simulink model "DDC_test"  (Simulink 7.4)
settings: Solver=ode3  StartTime=0.0  StopTime=Inf  FixedStep=1  RelTol=1e-3
undefined symbols (not defined in the file): Fs, get, j, sided, Two
libraries: simulink x6, dspsnks4 x5, dspsigops x2
settings Model: Creator=babjak  LastModifiedBy=babjak

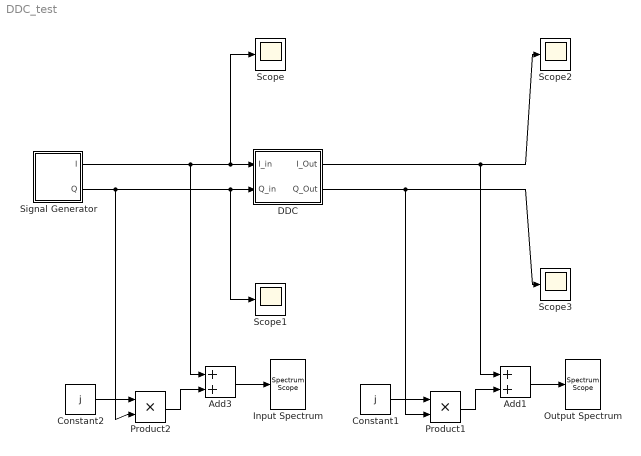
== system DDC_test ==
  Add1 : Sum  OutDataType=fixdt(1, 16)  OutScaling=2^-10
  Add3 : Sum  OutDataType=fixdt(1, 16)  OutScaling=2^-10
  Constant1 : Constant  Value=j  OutDataType=fixdt(1, 16)  OutScaling=2^0
  Constant2 : Constant  Value=j  OutDataType=fixdt(1, 16)  OutScaling=2^0
  DDC : Subsystem
  Input Spectrum : dspsnks4/Spectrum Scope  DialogController=dspdialog.SpectrumScope  DialogControllerArgs=DataTag3  SystemSampleTime=-1  ScopeProperties=on  Domain=Frequency  HorizSpan=1  UseBuffer=on  BufferSize=128  Overlap=0  inpFftLenInherit=off  FFTlength=128  numAvg=2  DisplayProperties=off  AxisGrid=on  Memory=off  FrameNumber=on  AxisLegend=off  AxisZoom=off  OpenScopeAtSimStart=on  OpenScopeImmediately=off  FigPos=get(0,'defaultfigureposition')  AxisProperties=off  XUnits=Hertz  XRange=Two-sided ((-Fs/2...Fs/2])  XDisplay=0  InheritXIncr=off  XIncr=3.6e-7  XLabel=Samples  XLimit=Auto  YUnits=dBW/Hertz  XMax=1  XMin=0  YLabel=Magnitude-squared, dB  LineProperties=off  wintypeSpecScope=Boxcar  RsSpecScope=50  betaSpecScope=5  winsampSpecScope=Periodic  XAxisParamsVer=6.9
      settings: YMin=-10  YMax=10
  Output Spectrum : dspsnks4/Spectrum Scope  DialogController=dspdialog.SpectrumScope  DialogControllerArgs=DataTag4  SystemSampleTime=-1  ScopeProperties=on  Domain=Frequency  HorizSpan=1  UseBuffer=on  BufferSize=128  Overlap=0  inpFftLenInherit=off  FFTlength=128  numAvg=2  DisplayProperties=off  AxisGrid=on  Memory=off  FrameNumber=on  AxisLegend=off  AxisZoom=off  OpenScopeAtSimStart=on  OpenScopeImmediately=off  FigPos=get(0,'defaultfigureposition')  AxisProperties=off  XUnits=Hertz  XRange=Two-sided ((-Fs/2...Fs/2])  XDisplay=0  InheritXIncr=off  XIncr=1.44e-6  XLabel=Samples  XLimit=Auto  YUnits=dBW/Hertz  XMax=1  XMin=0  YLabel=Magnitude-squared, dB  LineProperties=off  wintypeSpecScope=Boxcar  RsSpecScope=50  betaSpecScope=5  winsampSpecScope=Periodic  XAxisParamsVer=6.9
      settings: YMin=-10  YMax=10
  Product1 : Product  OutDataType=fixdt(1, 16)  OutScaling=2^0  RndMeth=Zero
  Product2 : Product  OutDataType=fixdt(1, 16)  OutScaling=2^0  RndMeth=Zero
  Scope{,1..3} (4 alike) : Scope
      Scope2 settings: SaveName=ScopeData2
      Scope3 settings: SaveName=ScopeData3
  Signal Generator : Subsystem
  wires:
  DDC/1(I_Out) -> Scope2/1, Add1/1
  DDC/2(Q_Out) -> Scope3/1, Product1/2
  Signal Generator/1(I) -> DDC/1(I_in), Scope/1, Add3/1
  Signal Generator/2(Q) -> DDC/2(Q_in), Scope1/1, Product2/2
  Constant2/1 -> Product2/1
  Product2/1 -> Add3/2
  Add3/1 -> Input Spectrum/1
  Constant1/1 -> Product1/1
  Product1/1 -> Add1/2
  Add1/1 -> Output Spectrum/1

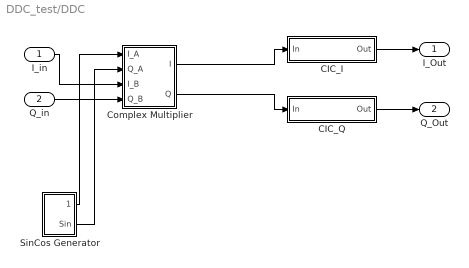
== system DDC_test/DDC ==
  I_in : Inport  DataType=Specify via dialog  OutDataType=fixdt(1,14,0)  OutDataTypeStr=fixdt(1,14,0)
  Q_in : Inport  Port=2  DataType=Specify via dialog  OutDataType=fixdt(1,14,0)  OutDataTypeStr=fixdt(1,14,0)
  CIC_I : Subsystem
  CIC_Q : Subsystem
  Complex Multiplier : Subsystem
  SinCos Generator : Subsystem
  I_Out : Outport
  Q_Out : Outport  Port=2
  wires:
  SinCos Generator/1(Cos) -> Complex Multiplier/1(I_A)
  SinCos Generator/2(Sin) -> Complex Multiplier/2(Q_A)
  Complex Multiplier/1(I) -> CIC_I/1(In)
  I_in/1 -> Complex Multiplier/3(I_B)
  Complex Multiplier/2(Q) -> CIC_Q/1(In)
  Q_in/1 -> Complex Multiplier/4(Q_B)
  CIC_I/1(Out) -> I_Out/1
  CIC_Q/1(Out) -> Q_Out/1

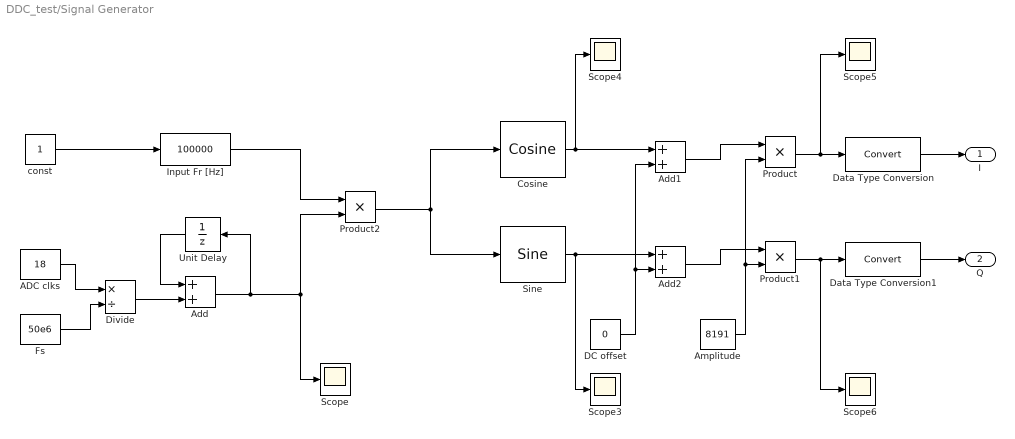
== system DDC_test/Signal Generator ==
  ADC clks : Constant  Value=18  OutDataTypeMode=double  OutDataType=fixdt(1,16)  ConRadixGroup=Best Precision: Vector-wise  OutDataTypeStr=double  SampleTime=Inf
  Add : Sum  OutDataTypeMode=double  OutDataTypeStr=double  SampleTime=1
  Add1 : Sum  OutDataType=fixdt(1, 16)  OutScaling=2^-10
  Add2 : Sum  OutDataType=fixdt(1, 16)  OutScaling=2^-10
  Amplitude : Constant  Value=8191  OutDataType=fixdt(1, 16)  OutScaling=2^0
  Cosine : simulink/Lookup Tables/Cosine  SystemSampleTime=-1  Formula=cos(2*pi*u)  NumDataPoints=(2^5)+1  OutputWordLength=8
  DC offset : Constant  Value=0  OutDataType=fixdt(1, 16)  OutScaling=2^0
  Data Type Conversion : DataTypeConversion  OutDataType=fixdt(1, 16)  OutScaling=2^0
  Data Type Conversion1 : DataTypeConversion  OutDataType=fixdt(1, 16)  OutScaling=2^0
  Divide : Product  Inputs=*/  OutDataTypeMode=double  OutDataType=fixdt(1, 16)  OutScaling=2^-10  OutDataTypeStr=double  SampleTime=1
  Fs : Constant  Value=50e6  OutDataTypeMode=double  OutDataType=fixdt(1,16)  ConRadixGroup=Best Precision: Vector-wise  OutDataTypeStr=double  SampleTime=Inf
  Input Fr [Hz] : simulink/Math Operations/Slider Gain  SystemSampleTime=-1  low=0  gain=100000  high=1500000
  Product : Product  OutDataType=fixdt(1, 16)  OutScaling=2^0  RndMeth=Zero
  Product1 : Product  OutDataType=fixdt(1, 16)  OutScaling=2^0  RndMeth=Zero
  Product2 : Product  OutDataTypeMode=double  OutDataType=fixdt(1, 16)  OutScaling=2^0  OutDataTypeStr=double  RndMeth=Zero
  Scope{,3..6} (5 alike) : Scope
      Scope settings: SaveName=ScopeData4
      Scope3 settings: SaveName=ScopeData7
      Scope4 settings: SaveName=ScopeData8
      Scope5 settings: SaveName=ScopeData9
      Scope6 settings: SaveName=ScopeData29
  Sine : simulink/Lookup Tables/Sine  SystemSampleTime=-1  Formula=sin(2*pi*u)  NumDataPoints=(2^5)+1  OutputWordLength=8
  Unit Delay : UnitDelay  SampleTime=-1
  const : Constant  OutDataTypeMode=double  OutDataType=fixdt(1,16)  ConRadixGroup=Best Precision: Vector-wise  OutDataTypeStr=double  SampleTime=Inf
  I : Outport  OutDataType=fixdt(1, 16)  OutScaling=2^0
  Q : Outport  Port=2  OutDataType=fixdt(1, 16)  OutScaling=2^0
  wires:
  Cosine/1 -> Add1/1, Scope4/1
  Sine/1 -> Add2/1, Scope3/1
  DC offset/1 -> Add1/2, Add2/2
  Add1/1 -> Product/1
  Add2/1 -> Product1/1
  Amplitude/1 -> Product/2, Product1/2
  Product/1 -> Data Type Conversion/1, Scope5/1
  Product1/1 -> Data Type Conversion1/1, Scope6/1
  Data Type Conversion1/1 -> Q/1
  Data Type Conversion/1 -> I/1
  Unit Delay/1 -> Add/1
  Add/1 -> Unit Delay/1, Product2/2, Scope/1
  Input Fr [Hz]/1 -> Product2/1
  Product2/1 -> Cosine/1, Sine/1
  ADC clks/1 -> Divide/1
  Fs/1 -> Divide/2
  Divide/1 -> Add/2
  const/1 -> Input Fr [Hz]/1

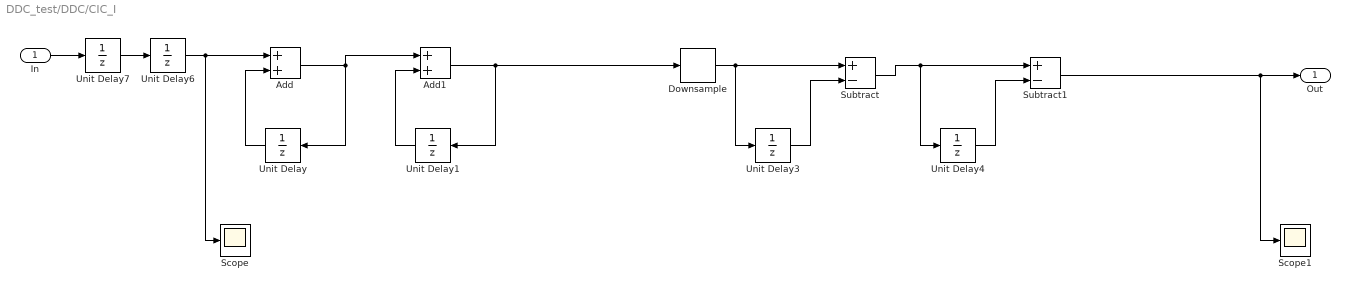
== system DDC_test/DDC/CIC_I ==
  In : Inport  SampleTime=1  OutDataType=fixdt(0,23,0)
  Add : Sum  OutDataTypeMode=Specify via dialog  OutDataType=fixdt(1,32,0)  OutDataTypeStr=fixdt(1,32,0)
  Add1 : Sum  OutDataTypeMode=Specify via dialog  OutDataType=fixdt(1,32,0)  OutDataTypeStr=fixdt(1,32,0)
  Downsample : dspsigops/Downsample  N=4  phase=0  ic=0  smode=Allow multirate  fmode=Maintain input frame size
  Scope : Scope
      settings: SaveName=ScopeData27
  Scope1 : Scope
      settings: SaveName=ScopeData28
  Subtract : Sum  Inputs=+-  OutDataTypeMode=Specify via dialog  OutDataType=fixdt(1,32,0)  OutDataTypeStr=fixdt(1,32,0)
  Subtract1 : Sum  Inputs=+-  OutDataTypeMode=Specify via dialog  OutDataType=fixdt(1,32,0)  OutDataTypeStr=fixdt(1,32,0)
  Unit Delay{,1,3..4,6..7} (6 alike) : UnitDelay  SampleTime=-1
  Out : Outport  OutDataType=fixdt(1, 16)  OutScaling=2^0
  wires:
  In/1 -> Unit Delay7/1
  Unit Delay/1 -> Add/2
  Add/1 -> Add1/1, Unit Delay/1
  Unit Delay1/1 -> Add1/2
  Add1/1 -> Unit Delay1/1, Downsample/1
  Unit Delay3/1 -> Subtract/2
  Downsample/1 -> Subtract/1, Unit Delay3/1
  Unit Delay4/1 -> Subtract1/2
  Subtract/1 -> Subtract1/1, Unit Delay4/1
  Subtract1/1 -> Out/1, Scope1/1
  Unit Delay6/1 -> Add/1, Scope/1
  Unit Delay7/1 -> Unit Delay6/1

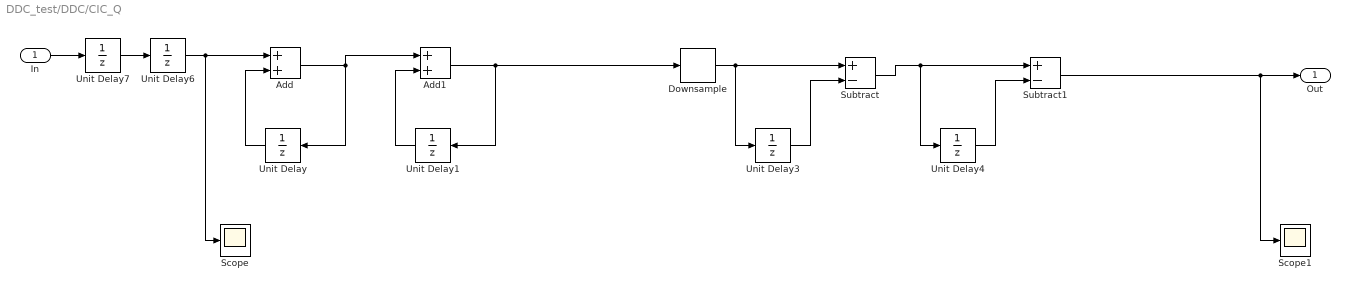
== system DDC_test/DDC/CIC_Q ==
  In : Inport  SampleTime=1  OutDataType=fixdt(0,23,0)
  Add : Sum  OutDataTypeMode=Specify via dialog  OutDataType=fixdt(1,32,0)  OutDataTypeStr=fixdt(1,32,0)
  Add1 : Sum  OutDataTypeMode=Specify via dialog  OutDataType=fixdt(1,32,0)  OutDataTypeStr=fixdt(1,32,0)
  Downsample : dspsigops/Downsample  N=4  phase=0  ic=0  smode=Allow multirate  fmode=Maintain input frame size
  Scope : Scope
      settings: SaveName=ScopeData5
  Scope1 : Scope
      settings: SaveName=ScopeData6
  Subtract : Sum  Inputs=+-  OutDataTypeMode=Specify via dialog  OutDataType=fixdt(1,32,0)  OutDataTypeStr=fixdt(1,32,0)
  Subtract1 : Sum  Inputs=+-  OutDataTypeMode=Specify via dialog  OutDataType=fixdt(1,32,0)  OutDataTypeStr=fixdt(1,32,0)
  Unit Delay{,1,3..4,6..7} (6 alike) : UnitDelay  SampleTime=-1
  Out : Outport  OutDataType=fixdt(1, 16)  OutScaling=2^0
  wires:
  In/1 -> Unit Delay7/1
  Unit Delay/1 -> Add/2
  Add/1 -> Add1/1, Unit Delay/1
  Unit Delay1/1 -> Add1/2
  Add1/1 -> Unit Delay1/1, Downsample/1
  Unit Delay3/1 -> Subtract/2
  Downsample/1 -> Subtract/1, Unit Delay3/1
  Unit Delay4/1 -> Subtract1/2
  Subtract/1 -> Subtract1/1, Unit Delay4/1
  Subtract1/1 -> Out/1, Scope1/1
  Unit Delay6/1 -> Add/1, Scope/1
  Unit Delay7/1 -> Unit Delay6/1

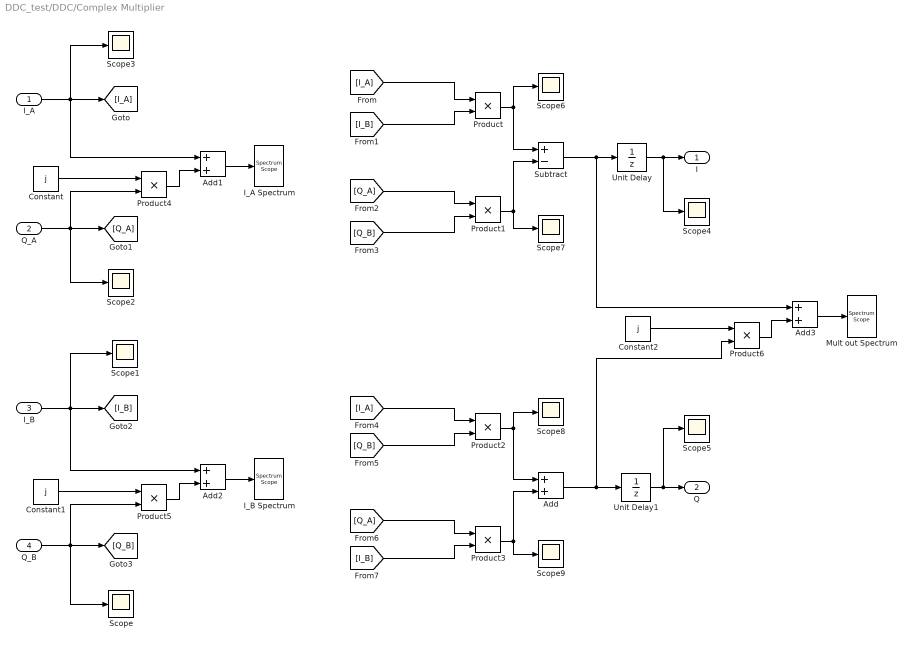
== system DDC_test/DDC/Complex Multiplier ==
  I_A : Inport  DataType=Specify via dialog  OutDataType=fixdt(1,8,0)  OutDataTypeStr=fixdt(1,8,0)
  Q_A : Inport  Port=2  DataType=Specify via dialog  OutDataType=fixdt(1,8,0)  OutDataTypeStr=fixdt(1,8,0)
  I_B : Inport  Port=3  DataType=Specify via dialog  OutDataType=fixdt(1,14,0)  OutDataTypeStr=fixdt(1,14,0)
  Q_B : Inport  Port=4  DataType=Specify via dialog  OutDataType=fixdt(1,14,0)  OutDataTypeStr=fixdt(1,14,0)
  Add : Sum  OutDataTypeMode=Specify via dialog  OutDataType=fixdt(1,23,0)  OutDataTypeStr=fixdt(1,23,0)
  Add1 : Sum  OutDataType=fixdt(1, 16)  OutScaling=2^-10
  Add2 : Sum  OutDataType=fixdt(1, 16)  OutScaling=2^-10
  Add3 : Sum  OutDataType=fixdt(1, 16)  OutScaling=2^-10
  Constant : Constant  Value=j  OutDataType=fixdt(1, 16)  OutScaling=2^0
  Constant1 : Constant  Value=j  OutDataType=fixdt(1, 16)  OutScaling=2^0
  Constant2 : Constant  Value=j  OutDataType=fixdt(1, 16)  OutScaling=2^0
  I_A Spectrum : dspsnks4/Spectrum Scope  DialogController=dspdialog.SpectrumScope  DialogControllerArgs=DataTag0  SystemSampleTime=-1  ScopeProperties=on  Domain=Frequency  HorizSpan=1  UseBuffer=on  BufferSize=128  Overlap=0  inpFftLenInherit=off  FFTlength=128  numAvg=1  DisplayProperties=off  AxisGrid=on  Memory=off  FrameNumber=on  AxisLegend=off  AxisZoom=off  OpenScopeAtSimStart=on  OpenScopeImmediately=off  FigPos=get(0,'defaultfigureposition')  AxisProperties=off  XUnits=Hertz  XRange=Two-sided ((-Fs/2...Fs/2])  XDisplay=0  InheritXIncr=off  XIncr=3.6e-7  XLabel=Samples  XLimit=Auto  YUnits=dBW/Hertz  XMax=1  XMin=0  YLabel=Magnitude-squared, dB  LineProperties=off  wintypeSpecScope=Boxcar  RsSpecScope=50  betaSpecScope=5  winsampSpecScope=Periodic  XAxisParamsVer=6.9
      settings: YMin=-10  YMax=10
  I_B Spectrum : dspsnks4/Spectrum Scope  DialogController=dspdialog.SpectrumScope  DialogControllerArgs=DataTag1  SystemSampleTime=-1  ScopeProperties=on  Domain=Frequency  HorizSpan=1  UseBuffer=on  BufferSize=128  Overlap=0  inpFftLenInherit=off  FFTlength=128  numAvg=1  DisplayProperties=off  AxisGrid=on  Memory=off  FrameNumber=on  AxisLegend=off  AxisZoom=off  OpenScopeAtSimStart=on  OpenScopeImmediately=off  FigPos=get(0,'defaultfigureposition')  AxisProperties=off  XUnits=Hertz  XRange=Two-sided ((-Fs/2...Fs/2])  XDisplay=0  InheritXIncr=off  XIncr=3.6e-7  XLabel=Samples  XLimit=Auto  YUnits=dBW/Hertz  XMax=1  XMin=0  YLabel=Magnitude-squared, dB  LineProperties=off  wintypeSpecScope=Boxcar  RsSpecScope=50  betaSpecScope=5  winsampSpecScope=Periodic  XAxisParamsVer=6.9
      settings: YMin=-10  YMax=10
  Mult out Spectrum : dspsnks4/Spectrum Scope  DialogController=dspdialog.SpectrumScope  DialogControllerArgs=DataTag2  SystemSampleTime=-1  ScopeProperties=on  Domain=Frequency  HorizSpan=1  UseBuffer=on  BufferSize=128  Overlap=0  inpFftLenInherit=off  FFTlength=128  numAvg=1  DisplayProperties=off  AxisGrid=on  Memory=off  FrameNumber=on  AxisLegend=off  AxisZoom=off  OpenScopeAtSimStart=on  OpenScopeImmediately=off  FigPos=get(0,'defaultfigureposition')  AxisProperties=off  XUnits=Hertz  XRange=Two-sided ((-Fs/2...Fs/2])  XDisplay=0  InheritXIncr=off  XIncr=3.6e-7  XLabel=Samples  XLimit=Auto  YUnits=dBW/Hertz  XMax=1  XMin=0  YLabel=Magnitude-squared, dB  LineProperties=off  wintypeSpecScope=Boxcar  RsSpecScope=50  betaSpecScope=5  winsampSpecScope=Periodic  XAxisParamsVer=6.9
      settings: YMin=-10  YMax=10
  Product{,1..3} (4 alike) : Product  OutDataTypeMode=Specify via dialog  OutDataType=fixdt(1,22,0)  OutDataTypeStr=fixdt(1,22,0)  RndMeth=Zero
  Product4 : Product  OutDataType=fixdt(1, 16)  OutScaling=2^0  RndMeth=Zero
  Product5 : Product  OutDataType=fixdt(1, 16)  OutScaling=2^0  RndMeth=Zero
  Product6 : Product  OutDataType=fixdt(1, 16)  OutScaling=2^0  RndMeth=Zero
  Scope{,1..9} (10 alike) : Scope
      Scope settings: YMin=-150  YMax=125  SaveName=ScopeData17
      Scope1 settings: YMin=-150  YMax=75  SaveName=ScopeData18
      Scope2 settings: YMin=-150  YMax=150  SaveName=ScopeData19
      Scope3 settings: YMin=-150  YMax=125  SaveName=ScopeData20
      Scope4 settings: YMin=-1.25e+006  YMax=1.25e+006  SaveName=ScopeData21
      Scope5 settings: YMin=-1.25e+006  YMax=1.25e+006  SaveName=ScopeData22
      Scope6 settings: YMin=-900000  YMax=100000  SaveName=ScopeData23
      Scope7 settings: YMin=0  YMax=900000  SaveName=ScopeData24
      Scope8 settings: YMin=-1e+006  YMax=500000  SaveName=ScopeData25
      Scope9 settings: YMin=-900000  YMax=400000  SaveName=ScopeData26
  Subtract : Sum  Inputs=+-  OutDataTypeMode=Specify via dialog  OutDataType=fixdt(1,23,0)  OutDataTypeStr=fixdt(1,23,0)
  Unit Delay : UnitDelay  SampleTime=-1
  Unit Delay1 : UnitDelay  SampleTime=-1
  I : Outport  OutDataType=fixdt(1, 16)  OutScaling=2^0
  Q : Outport  Port=2  OutDataType=fixdt(1, 16)  OutScaling=2^0
  wires:
  Product/1 -> Subtract/1, Scope6/1
  Subtract/1 -> Add3/1, Unit Delay/1
  Product1/1 -> Subtract/2, Scope7/1
  [I_A] -> Product2/1
  Product2/1 -> Add/1, Scope8/1
  [Q_B] -> Product2/2
  Add/1 -> Product6/2, Unit Delay1/1
  [Q_A] -> Product3/1
  Product3/1 -> Add/2, Scope9/1
  [I_B] -> Product3/2
  I_A/1 -> [I_A], Scope3/1, Add1/1
  Q_A/1 -> [Q_A], Scope2/1, Product4/2
  I_B/1 -> [I_B], Scope1/1, Add2/1
  Q_B/1 -> [Q_B], Scope/1, Product5/2
  [I_A] -> Product/1
  [I_B] -> Product/2
  [Q_A] -> Product1/1
  [Q_B] -> Product1/2
  Unit Delay/1 -> I/1, Scope4/1
  Unit Delay1/1 -> Q/1, Scope5/1
  Constant/1 -> Product4/1
  Product4/1 -> Add1/2
  Add1/1 -> I_A Spectrum/1
  Constant1/1 -> Product5/1
  Product5/1 -> Add2/2
  Add2/1 -> I_B Spectrum/1
  Constant2/1 -> Product6/1
  Product6/1 -> Add3/2
  Add3/1 -> Mult out Spectrum/1

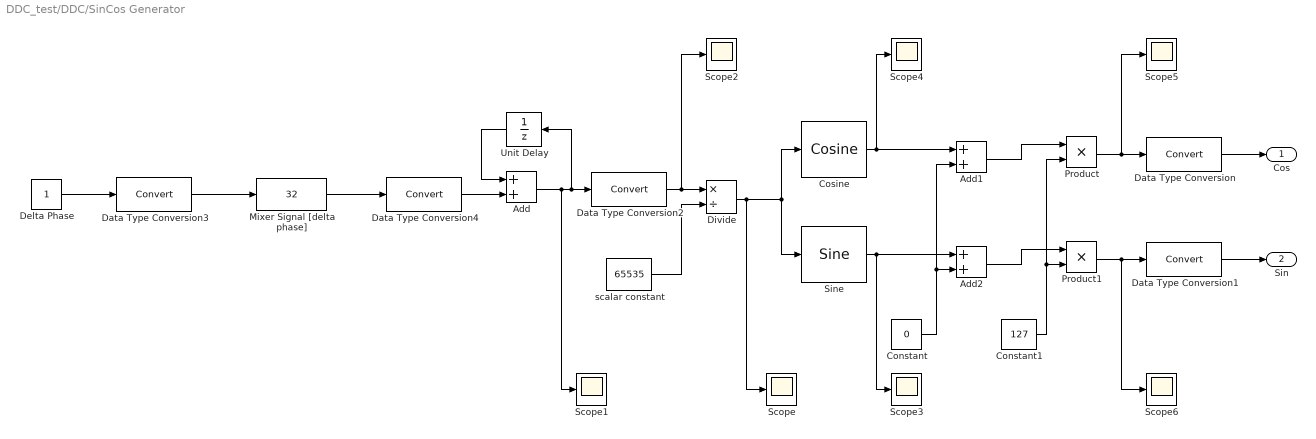
== system DDC_test/DDC/SinCos Generator ==
  Add : Sum  OutDataTypeMode=Specify via dialog  OutDataTypeStr=fixdt(1,16,0)  SampleTime=1
  Add1 : Sum  OutDataType=fixdt(1, 16)  OutScaling=2^-10
  Add2 : Sum  OutDataType=fixdt(1, 16)  OutScaling=2^-10
  Constant : Constant  Value=0  OutDataType=fixdt(1, 16)  OutScaling=2^0
  Constant1 : Constant  Value=127  OutDataType=fixdt(1, 16)  OutScaling=2^0
  Cosine : simulink/Lookup Tables/Cosine  SystemSampleTime=-1  Formula=cos(2*pi*u)  NumDataPoints=(2^5)+1  OutputWordLength=8
  Data Type Conversion{,1..4} (5 alike) : DataTypeConversion  OutDataType=fixdt(1, 16)  OutScaling=2^0
  Delta Phase : Constant  OutDataTypeMode=Specify via dialog  OutDataType=fixdt(1,16)  ConRadixGroup=Best Precision: Vector-wise  OutDataTypeStr=fixdt(1,16)  SampleTime=Inf
  Divide : Product  Inputs=*/  OutDataTypeMode=double  OutDataType=fixdt(1, 16)  OutScaling=2^-10  OutDataTypeStr=double  SampleTime=1
  Mixer Signal [delta phase] : simulink/Math Operations/Slider Gain  SystemSampleTime=-1  low=0  gain=32  high=1000
  Product : Product  OutDataType=fixdt(1, 16)  OutScaling=2^0  RndMeth=Zero
  Product1 : Product  OutDataType=fixdt(1, 16)  OutScaling=2^0  RndMeth=Zero
  Scope{,1..6} (7 alike) : Scope
      Scope settings: SaveName=ScopeData10
      Scope1 settings: SaveName=ScopeData11
      Scope2 settings: SaveName=ScopeData12
      Scope3 settings: SaveName=ScopeData13
      Scope4 settings: SaveName=ScopeData14
      Scope5 settings: SaveName=ScopeData15
      Scope6 settings: SaveName=ScopeData16
  Sine : simulink/Lookup Tables/Sine  SystemSampleTime=-1  Formula=sin(2*pi*u)  NumDataPoints=(2^5)+1  OutputWordLength=8
  Unit Delay : UnitDelay  SampleTime=-1
  scalar constant : Constant  Value=65535  OutDataTypeMode=double  OutDataType=fixdt(1,16)  ConRadixGroup=Best Precision: Vector-wise  OutDataTypeStr=double  SampleTime=Inf
  Cos : Outport  OutDataType=fixdt(1, 16)  OutScaling=2^0
  Sin : Outport  Port=2  OutDataType=fixdt(1, 16)  OutScaling=2^0
  wires:
  Add/1 -> Unit Delay/1, Data Type Conversion2/1, Scope1/1
  Delta Phase/1 -> Data Type Conversion3/1
  scalar constant/1 -> Divide/2
  Divide/1 -> Sine/1, Cosine/1, Scope/1
  Cosine/1 -> Add1/1, Scope4/1
  Sine/1 -> Add2/1, Scope3/1
  Constant/1 -> Add1/2, Add2/2
  Add1/1 -> Product/1
  Add2/1 -> Product1/1
  Constant1/1 -> Product/2, Product1/2
  Product/1 -> Data Type Conversion/1, Scope5/1
  Product1/1 -> Data Type Conversion1/1, Scope6/1
  Data Type Conversion1/1 -> Sin/1
  Data Type Conversion/1 -> Cos/1
  Unit Delay/1 -> Add/1
  Data Type Conversion2/1 -> Divide/1, Scope2/1
  Mixer Signal [delta phase]/1 -> Data Type Conversion4/1
  Data Type Conversion3/1 -> Mixer Signal [delta phase]/1
  Data Type Conversion4/1 -> Add/2
